simulink model "comparation_models"  (R2022b)
settings: Solver=VariableStepAuto  StartTime=0.0  StopTime=t_sample*n_sample  RelTol=1e-3
values from neighbouring files (symbols this model uses):
  air_den = 1.225    [wind_turbine_parameters.m]
  l1 = 56    [wind_turbine_parameters.m]
  lambda_op = 5.68    [wind_turbine_parameters.m]
undefined symbols (not defined in the file or in its folder): pitch_deg, t_sample2
libraries: simulink x1
settings Model: Creator=marina  LastModifiedBy=marina

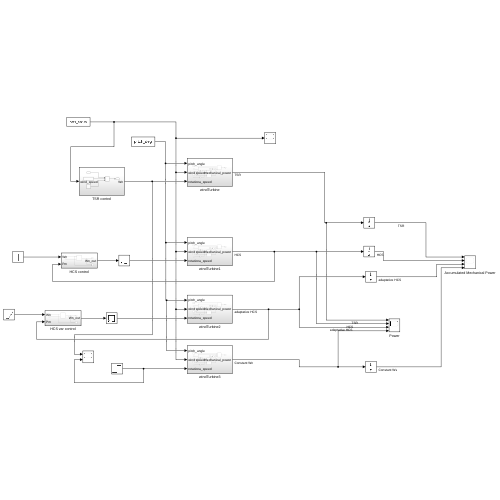
[thumbnail: Simulink's stored preview of the top-level diagram]
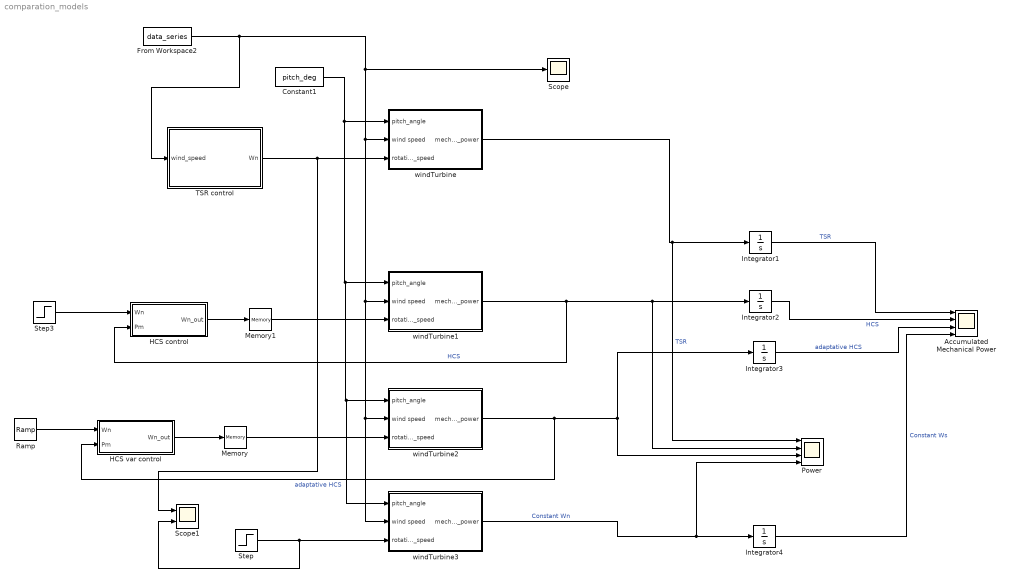
== system comparation_models ==
  Accumulated Mechanical Power : Scope  NumInputPorts=4
  Constant1 : Constant  Value=pitch_deg
  From Workspace2 : FromWorkspace  VariableName=data_series  SampleTime=t_sample2  OutputAfterFinalValue=Holding final value
  HCS control : Subsystem
  HCS var control : Subsystem
  Integrator{1..4} (4 alike) : Integrator
  Memory : Memory
  Memory1 : Memory
  Power : Scope  NumInputPorts=4
  Ramp : simulink/Sources/Ramp  slope=0.000007  start=0  InitialOutput=0.0001
  Scope : Scope
  Scope1 : Scope  NumInputPorts=2
  Step : Step  Time=0  After=0.9  SampleTime=0
  Step3 : Step  Time=0  SampleTime=0
  TSR control : Subsystem
  windTurbine : Subsystem
  windTurbine1 : Subsystem
  windTurbine2 : Subsystem
  windTurbine3 : Subsystem
  wires:
  TSR control/1(Wn) -> Scope1/1, windTurbine/3(rotationa_speed)
  From Workspace2/1 -> TSR control/1(wind_speed), Scope/1, windTurbine3/2(wind speed), windTurbine2/2(wind speed), windTurbine1/2(wind speed), windTurbine/2(wind speed)
  Integrator1/1 -> Accumulated Mechanical Power/1  "TSR"
  windTurbine/1(mechanical_power) -> Power/1, Integrator1/1  "TSR"
  Integrator2/1 -> Accumulated Mechanical Power/2  "HCS"
  Integrator3/1 -> Accumulated Mechanical Power/3  "adaptative HCS"
  windTurbine1/1(mechanical_power) -> HCS control/2(Pm), Power/2, Integrator2/1  "HCS"
  windTurbine2/1(mechanical_power) -> HCS var control/2(Pm), Integrator3/1, Power/3  "adaptative HCS"
  Constant1/1 -> windTurbine3/1(pitch_angle), windTurbine2/1(pitch_angle), windTurbine1/1(pitch_angle), windTurbine/1(pitch_angle)
  HCS var control/1(Wn_out) -> Memory/1
  Memory/1 -> windTurbine2/3(rotationa_speed)
  Ramp/1 -> HCS var control/1(Wn)
  HCS control/1(Wn_out) -> Memory1/1
  Memory1/1 -> windTurbine1/3(rotationa_speed)
  Step3/1 -> HCS control/1(Wn)
  windTurbine3/1(mechanical_power) -> Power/4, Integrator4/1  "Constant Wn"
  Step/1 -> Scope1/2, windTurbine3/3(rotationa_speed)
  Integrator4/1 -> Accumulated Mechanical Power/4  "Constant Ws"

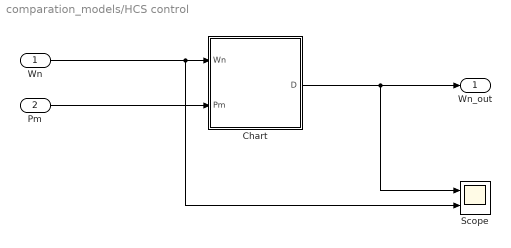
== system comparation_models/HCS control ==
  Wn : Inport
  Pm : Inport  Port=2
  Chart : Stateflow chart  TreatAsAtomicUnit=on
  Scope : Scope  NumInputPorts=2
  Wn_out : Outport
  wires:
  Pm/1 -> Chart/2(Pm)
  Wn/1 -> Scope/2, Chart/1(Wn)
  Chart/1(D) -> Scope/1, Wn_out/1

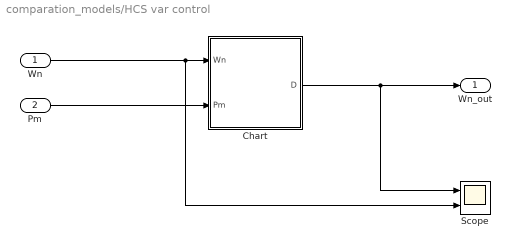
== system comparation_models/HCS var control ==
  Wn : Inport
  Pm : Inport  Port=2
  Chart : Stateflow chart  TreatAsAtomicUnit=on
  Scope : Scope  NumInputPorts=2
  Wn_out : Outport
  wires:
  Pm/1 -> Chart/2(Pm)
  Wn/1 -> Scope/2, Chart/1(Wn)
  Chart/1(D) -> Scope/1, Wn_out/1

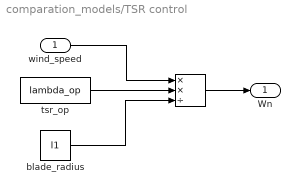
== system comparation_models/TSR control ==
  wind_speed : Inport
  " " : Product  Inputs=**/
  blade_radius : Constant  Value=l1
  tsr_op : Constant  Value=lambda_op
  Wn : Outport
  wires:
  " "/1 -> Wn/1
  tsr_op/1 -> " "/2
  wind_speed/1 -> " "/1
  blade_radius/1 -> " "/3

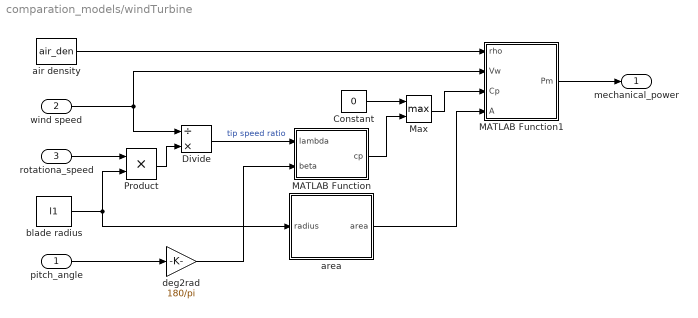
== system comparation_models/windTurbine ==
  pitch_angle : Inport
  wind speed : Inport  Port=2
  rotationa_speed : Inport  Port=3
  Constant : Constant  Value=0
  Divide : Product  Inputs=/*
  MATLAB Function : MATLAB Function  TreatAsAtomicUnit=on
  MATLAB Function1 : MATLAB Function  TreatAsAtomicUnit=on
  Max : MinMax  Function=max  Inputs=2
  Product : Product
  air density : Constant  Value=air_den
  area : Subsystem
  blade radius : Constant  Value=l1
  deg2rad : Gain  Gain=180/pi
  mechanical_power : Outport
  wires:
  Product/1 -> Divide/2
  wind speed/1 -> Divide/1, MATLAB Function1/2(Vw)
  Divide/1 -> MATLAB Function/1(lambda)  "tip speed ratio"
  pitch_angle/1 -> deg2rad/1
  MATLAB Function1/1(Pm) -> mechanical_power/1
  rotationa_speed/1 -> Product/1
  air density/1 -> MATLAB Function1/1(rho)
  area/1(area) -> MATLAB Function1/4(A)
  blade radius/1 -> Product/2, area/1(radius)
  deg2rad/1 -> MATLAB Function/2(beta)
  Max/1 -> MATLAB Function1/3(Cp)
  MATLAB Function/1(cp) -> Max/2
  Constant/1 -> Max/1

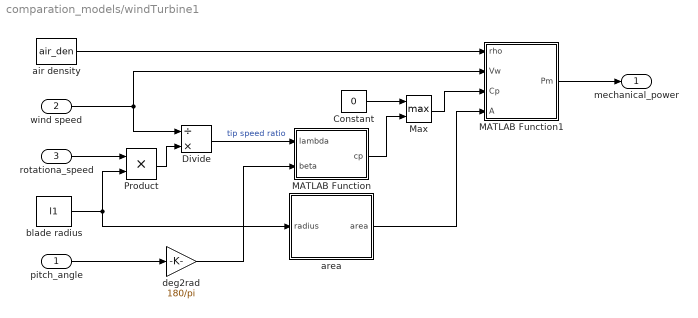
== system comparation_models/windTurbine1 ==
  pitch_angle : Inport
  wind speed : Inport  Port=2
  rotationa_speed : Inport  Port=3
  Constant : Constant  Value=0
  Divide : Product  Inputs=/*
  MATLAB Function : MATLAB Function  TreatAsAtomicUnit=on
  MATLAB Function1 : MATLAB Function  TreatAsAtomicUnit=on
  Max : MinMax  Function=max  Inputs=2
  Product : Product
  air density : Constant  Value=air_den
  area : Subsystem
  blade radius : Constant  Value=l1
  deg2rad : Gain  Gain=180/pi
  mechanical_power : Outport
  wires:
  Product/1 -> Divide/2
  wind speed/1 -> Divide/1, MATLAB Function1/2(Vw)
  Divide/1 -> MATLAB Function/1(lambda)  "tip speed ratio"
  pitch_angle/1 -> deg2rad/1
  MATLAB Function1/1(Pm) -> mechanical_power/1
  rotationa_speed/1 -> Product/1
  air density/1 -> MATLAB Function1/1(rho)
  area/1(area) -> MATLAB Function1/4(A)
  blade radius/1 -> Product/2, area/1(radius)
  deg2rad/1 -> MATLAB Function/2(beta)
  Max/1 -> MATLAB Function1/3(Cp)
  MATLAB Function/1(cp) -> Max/2
  Constant/1 -> Max/1

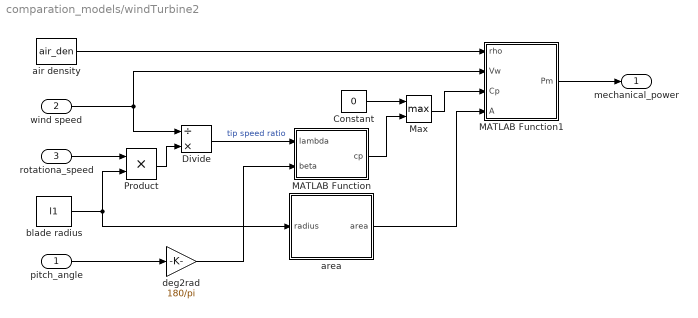
== system comparation_models/windTurbine2 ==
  pitch_angle : Inport
  wind speed : Inport  Port=2
  rotationa_speed : Inport  Port=3
  Constant : Constant  Value=0
  Divide : Product  Inputs=/*
  MATLAB Function : MATLAB Function  TreatAsAtomicUnit=on
  MATLAB Function1 : MATLAB Function  TreatAsAtomicUnit=on
  Max : MinMax  Function=max  Inputs=2
  Product : Product
  air density : Constant  Value=air_den
  area : Subsystem
  blade radius : Constant  Value=l1
  deg2rad : Gain  Gain=180/pi
  mechanical_power : Outport
  wires:
  Product/1 -> Divide/2
  wind speed/1 -> Divide/1, MATLAB Function1/2(Vw)
  Divide/1 -> MATLAB Function/1(lambda)  "tip speed ratio"
  pitch_angle/1 -> deg2rad/1
  MATLAB Function1/1(Pm) -> mechanical_power/1
  rotationa_speed/1 -> Product/1
  air density/1 -> MATLAB Function1/1(rho)
  area/1(area) -> MATLAB Function1/4(A)
  blade radius/1 -> Product/2, area/1(radius)
  deg2rad/1 -> MATLAB Function/2(beta)
  Max/1 -> MATLAB Function1/3(Cp)
  MATLAB Function/1(cp) -> Max/2
  Constant/1 -> Max/1

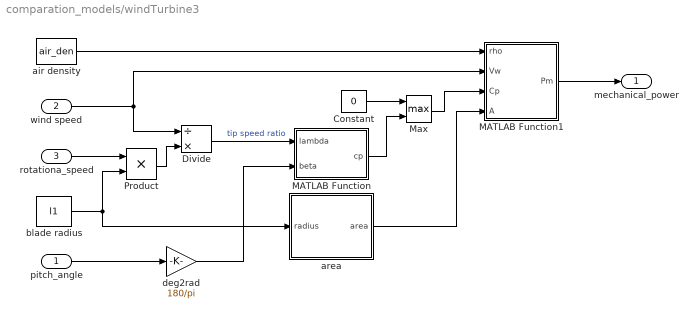
== system comparation_models/windTurbine3 ==
  pitch_angle : Inport
  wind speed : Inport  Port=2
  rotationa_speed : Inport  Port=3
  Constant : Constant  Value=0
  Divide : Product  Inputs=/*
  MATLAB Function : MATLAB Function  TreatAsAtomicUnit=on
  MATLAB Function1 : MATLAB Function  TreatAsAtomicUnit=on
  Max : MinMax  Function=max  Inputs=2
  Product : Product
  air density : Constant  Value=air_den
  area : Subsystem
  blade radius : Constant  Value=l1
  deg2rad : Gain  Gain=180/pi
  mechanical_power : Outport
  wires:
  Product/1 -> Divide/2
  wind speed/1 -> Divide/1, MATLAB Function1/2(Vw)
  Divide/1 -> MATLAB Function/1(lambda)  "tip speed ratio"
  pitch_angle/1 -> deg2rad/1
  MATLAB Function1/1(Pm) -> mechanical_power/1
  rotationa_speed/1 -> Product/1
  air density/1 -> MATLAB Function1/1(rho)
  area/1(area) -> MATLAB Function1/4(A)
  blade radius/1 -> Product/2, area/1(radius)
  deg2rad/1 -> MATLAB Function/2(beta)
  Max/1 -> MATLAB Function1/3(Cp)
  MATLAB Function/1(cp) -> Max/2
  Constant/1 -> Max/1

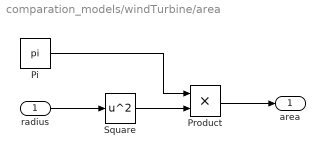
== system comparation_models/windTurbine/area ==
  radius : Inport
  Pi : Constant  Value=pi  OutDataTypeStr=Inherit: Inherit via back propagation
  Product : Product
  Square : Math  Operator=square
  area : Outport
  wires:
  radius/1 -> Square/1
  Square/1 -> Product/2
  Pi/1 -> Product/1
  Product/1 -> area/1

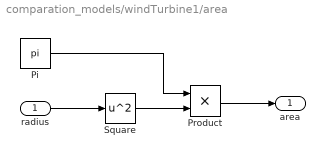
== system comparation_models/windTurbine1/area ==
  radius : Inport
  Pi : Constant  Value=pi  OutDataTypeStr=Inherit: Inherit via back propagation
  Product : Product
  Square : Math  Operator=square
  area : Outport
  wires:
  radius/1 -> Square/1
  Square/1 -> Product/2
  Pi/1 -> Product/1
  Product/1 -> area/1

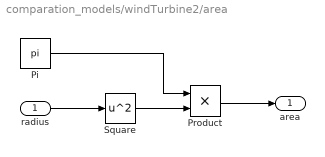
== system comparation_models/windTurbine2/area ==
  radius : Inport
  Pi : Constant  Value=pi  OutDataTypeStr=Inherit: Inherit via back propagation
  Product : Product
  Square : Math  Operator=square
  area : Outport
  wires:
  radius/1 -> Square/1
  Square/1 -> Product/2
  Pi/1 -> Product/1
  Product/1 -> area/1

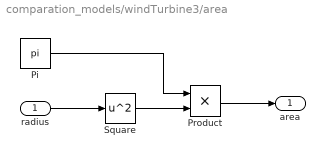
== system comparation_models/windTurbine3/area ==
  radius : Inport
  Pi : Constant  Value=pi  OutDataTypeStr=Inherit: Inherit via back propagation
  Product : Product
  Square : Math  Operator=square
  area : Outport
  wires:
  radius/1 -> Square/1
  Square/1 -> Product/2
  Pi/1 -> Product/1
  Product/1 -> area/1

== stateflow chart comparation_models/HCS control/Chart ==
  state stationary
    entry:
    D = Wn;
  state init_
    entry:
    D = Wn;
    pt_1 = 0;
    d_ = d;
  state measure
    entry:
    dp = Pm - pt_1;
    pt_1 = Pm;
  state decrease
    entry:
    d_ = - d_;
  state increase
    entry:
    d_ = d_;
  state perturb_
    entry:
    D = D + d_;
  measure -> stationary [order 3] : [abs(dp)< 500]
  stationary -> measure : [after(delay,sec)]
  (default) -> init_
  measure -> decrease [order 2] : [dp < 0]
  init_ -> measure
  perturb_ -> measure : [after(delay,sec)]
  decrease -> perturb_
  measure -> increase [order 1] : [dp > 0]
  increase -> perturb_
  data: Wn input; Pm input; D output; delay constant double =5; d constant double =0.05; pt_1 local; dp local; d_ local

== matlab function comparation_models/windTurbine3/MATLAB Function ==
  data: lambda input; cp output; beta input
function cp = fcn(lambda, beta)

k = load('coefficients.mat');
lambda_i =  1/(1/(lambda + 0.08*beta) - 0.035/(1+beta*beta*beta));

% Debug
% lambda_i
% k.k1 *(k.k2/lambda_i - k.k3*beta - k.k4*power(beta, k.k5) -k.k6)*exp(-k.k7/lambda_i)

cp = k.k1 *(k.k2/lambda_i - k.k3*beta - k.k4*power(beta, k.k5) -k.k6)*exp(-k.k7/lambda_i);

== matlab function comparation_models/windTurbine3/MATLAB Function1 ==
  data: rho input; Vw input; Pm output; Cp input; A input
function Pm = fcn(rho, Vw, Cp, A)

Pm = 0.5* Cp* rho* A* power(Vw, 3);

== matlab function comparation_models/windTurbine1/MATLAB Function ==
  data: lambda input; cp output; beta input
function cp = fcn(lambda, beta)

k = load('coefficients.mat');
lambda_i =  1/(1/(lambda + 0.08*beta) - 0.035/(1+beta*beta*beta));

% Debug
% lambda_i
% k.k1 *(k.k2/lambda_i - k.k3*beta - k.k4*power(beta, k.k5) -k.k6)*exp(-k.k7/lambda_i)

cp = k.k1 *(k.k2/lambda_i - k.k3*beta - k.k4*power(beta, k.k5) -k.k6)*exp(-k.k7/lambda_i);

== matlab function comparation_models/windTurbine1/MATLAB Function1 ==
  data: rho input; Vw input; Pm output; Cp input; A input
function Pm = fcn(rho, Vw, Cp, A)

Pm = 0.5* Cp* rho* A* power(Vw, 3);

== matlab function comparation_models/windTurbine/MATLAB Function ==
  data: lambda input; cp output; beta input
function cp = fcn(lambda, beta)

k = load('coefficients.mat');
lambda_i =  1/(1/(lambda + 0.08*beta) - 0.035/(1+beta*beta*beta));

% Debug
% lambda_i
% k.k1 *(k.k2/lambda_i - k.k3*beta - k.k4*power(beta, k.k5) -k.k6)*exp(-k.k7/lambda_i)

cp = k.k1 *(k.k2/lambda_i - k.k3*beta - k.k4*power(beta, k.k5) -k.k6)*exp(-k.k7/lambda_i);

== matlab function comparation_models/windTurbine/MATLAB Function1 ==
  data: rho input; Vw input; Pm output; Cp input; A input
function Pm = fcn(rho, Vw, Cp, A)

Pm = 0.5* Cp* rho* A* power(Vw, 3);

== matlab function comparation_models/windTurbine2/MATLAB Function ==
  data: lambda input; cp output; beta input
function cp = fcn(lambda, beta)

k = load('coefficients.mat');
lambda_i =  1/(1/(lambda + 0.08*beta) - 0.035/(1+beta*beta*beta));

% Debug
% lambda_i
% k.k1 *(k.k2/lambda_i - k.k3*beta - k.k4*power(beta, k.k5) -k.k6)*exp(-k.k7/lambda_i)

cp = k.k1 *(k.k2/lambda_i - k.k3*beta - k.k4*power(beta, k.k5) -k.k6)*exp(-k.k7/lambda_i);

== matlab function comparation_models/windTurbine2/MATLAB Function1 ==
  data: rho input; Vw input; Pm output; Cp input; A input
function Pm = fcn(rho, Vw, Cp, A)

Pm = 0.5* Cp* rho* A* power(Vw, 3);

== stateflow chart comparation_models/HCS var control/Chart ==
  state stationary
    entry:
    D = Wn;
  state init_
    entry:
    D = Wn;
    pt_1 = 0;
    d_ = d;
  state measure
    entry:
    dp = Pm - pt_1;
    pt_1 = Pm;
  state decrease
    entry:
    d_ = - d_;
  state increase
    entry:
    d_ = d_;
  state perturb_
    entry:
    D = D + d_;
  measure -> stationary [order 3] : [abs(dp)< 500]
  stationary -> measure : [after(delay,sec)]
  (default) -> init_
  measure -> decrease [order 2] : [dp < 0]
  init_ -> measure
  perturb_ -> measure : [after(delay,sec)]
  decrease -> perturb_
  measure -> increase [order 1] : [dp > 0]
  increase -> perturb_
  data: Wn input; Pm input; D output; delay constant double =5; d constant double =0.05; pt_1 local; dp local; d_ local
